simulink model "SimplifiedSystem"  (R2024b)
settings: Solver=VariableStepAuto  StartTime=0.0  StopTime=10.0  RelTol=1e-3
InitFcn:
  | Design
values from neighbouring files (symbols this model uses):
  Kd = Kp * Td    [DesignPIDBode.m]
  Ki = Kp / Ti    [DesignPIDBode.m]
  Kp = deltaK * cos(deltaPhi)    [DesignPIDBode.m]
  Ref = 50    [Design.m]
  Tl = 1/(5*Wgc)    [DesignPIDBode.m]
undefined symbols (not defined in the file or in its folder): daq, SS
libraries: simulink_extras x2
settings Model: Creator=Banaan  LastModifiedBy=Banaan

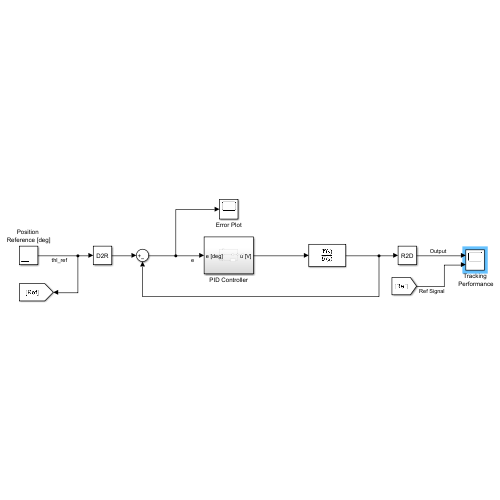
[thumbnail: Simulink's stored preview of the top-level diagram]
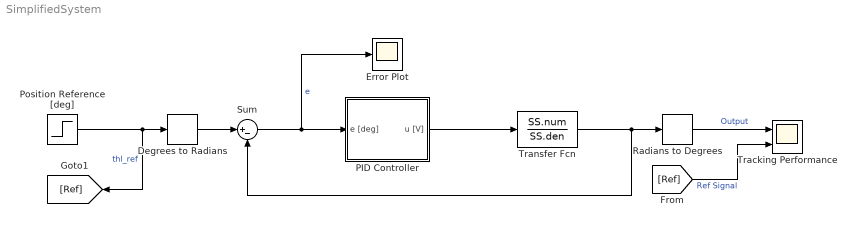
== system SimplifiedSystem ==
  Degrees to Radians : simulink_extras/Transformations/Degrees to Radians
  Error Plot : Scope
  PID Controller : Subsystem
  Position Reference [deg] : Step  After=Ref  SampleTime=0
  Radians to Degrees : simulink_extras/Transformations/Radians to Degrees
  Sum : Sum  Inputs=|+-
  Tracking Performance : Scope  NumInputPorts=2
  Transfer Fcn : TransferFcn  Numerator=SS.num  Denominator=SS.den
  wires:
  Transfer Fcn/1 -> Radians to Degrees/1, Sum/2
  Sum/1 -> Error Plot/1, PID Controller/1(e [deg])  "e"
  PID Controller/1(u [V]) -> Transfer Fcn/1
  Position Reference [deg]/1 -> [Ref], Degrees to Radians/1  "thl_ref"
  Degrees to Radians/1 -> Sum/1
  [Ref] -> Tracking Performance/2  "Ref Signal"
  Radians to Degrees/1 -> Tracking Performance/1  "Output"

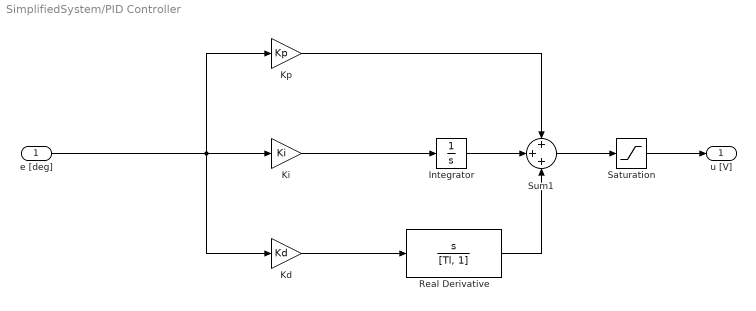
== system SimplifiedSystem/PID Controller ==
  e [deg] : Inport
  Integrator : Integrator
  Kd : Gain  Gain=Kd
  Ki : Gain  Gain=Ki
  Kp : Gain  Gain=Kp
  Real Derivative : TransferFcn  Numerator=[1, 0]  Denominator=[Tl, 1]
  Saturation : Saturate  UpperLimit=daq.adc.fs  LowerLimit=-daq.adc.fs
  Sum1 : Sum  Inputs=+++
  u [V] : Outport
  wires:
  e [deg]/1 -> Kd/1, Ki/1, Kp/1
  Real Derivative/1 -> Sum1/3
  Integrator/1 -> Sum1/2
  Kd/1 -> Real Derivative/1
  Ki/1 -> Integrator/1
  Kp/1 -> Sum1/1
  Sum1/1 -> Saturation/1
  Saturation/1 -> u [V]/1
